simulink model "JointSpaceControl_BestInertia"  (R2013a)
settings: Solver=ode3  StartTime=0.0  StopTime=sim_end  FixedStep=0.004  MaxStep=0.008  RelTol=1e-3
PreLoadFcn:
  | Initialization
InitFcn:
  | Initialization
values from neighbouring files (symbols this model uses):
  a_max = [27 27 27 27 27 27]    [Initialization.m]
  dq_0 = qd_actual.signals.values(1,:)    [Initialization.m]
  K_0 = [K0_11, zeros(3,3); zeros(3,3),omega_P_small^2*eye(3,3)]    [Initialization.m]    (also in Plot_PD_Estimation.m)
  K_1 = [K1_11, zeros(3,3); zeros(3,3),2*omega_D_small*eye(3,3)]    [Initialization.m]    (also in Plot_PD_Estimation.m)
  q_0 = q_actual.signals.values(1,:)    [Initialization.m]
  q_max = 2*pi*ones(1,6)    [Initialization.m]
  q_min = -2*pi*ones(1,6)    [Initialization.m]
  torque_max = [150 150 150 28 28 28]    [Initialization.m]
  v_max = 3.4*ones(1,6)    [Initialization.m]
libraries: dsparch4 x30, simulink x2
(part 3 of 3)

== matlab function JointSpaceControl_BestInertia/Forward & Velocity Kinematics Joint -> Tool Geometric Jacobian/J_a ==
  data: J_a output; q input; theta input; phi input; psi input
function J_a     = Analytical_Jacobian(q, theta, phi, psi)
% ANALYTICAL JACOBIAN - Jacobian from Base to Tool.
%  Calculates the analytical Jacobian, based on the Euler angle transform
%  representation.

theta_1 = q(1);
theta_2 = q(2);
theta_3 = q(3);
theta_4 = q(4);
theta_5 = q(5);
theta_6 = q(6);

J = [(109*cos(theta_1))/1000 + (41*cos(theta_1)*cos(theta_5))/500 + ...
        (17*cos(theta_2)*sin(theta_1))/40 - ...
        (93*cos(theta_4)*(cos(theta_2)*sin(theta_1)*sin(theta_3) + ...
        cos(theta_3)*sin(theta_1)*sin(theta_2)))/1000 + ...
        (93*sin(theta_4)*(sin(theta_1)*sin(theta_2)*sin(theta_3) - ...
        cos(theta_2)*cos(theta_3)*sin(theta_1)))/1000 - ...
        (41*sin(theta_5)*(cos(theta_4)*(sin(theta_1)*sin(theta_2)*sin(theta_3) - ...
        cos(theta_2)*cos(theta_3)*sin(theta_1)) + ...
        sin(theta_4)*(cos(theta_2)*sin(theta_1)*sin(theta_3) + ...
        cos(theta_3)*sin(theta_1)*sin(theta_2))))/500 - ...
        (39243*sin(theta_1)*sin(theta_2)*sin(theta_3))/100000 + ...
        (39243*cos(theta_2)*cos(theta_3)*sin(theta_1))/100000, ...
        ...
        (17*cos(theta_1)*sin(theta_2))/40 - ...
        (93*cos(theta_4)*(cos(theta_1)*sin(theta_2)*sin(theta_3) - ...
        cos(theta_1)*cos(theta_2)*cos(theta_3)))/1000 - ...
        (93*sin(theta_4)*(cos(theta_1)*cos(theta_2)*sin(theta_3) + ...
        cos(theta_1)*cos(theta_3)*sin(theta_2)))/1000 + ...
        (41*sin(theta_5)*(cos(theta_4)*(cos(theta_1)*cos(theta_2)*sin(theta_3) + ...
        cos(theta_1)*cos(theta_3)*sin(theta_2)) - ...
        sin(theta_4)*(cos(theta_1)*sin(theta_2)*sin(theta_3) - ...
        cos(theta_1)*cos(theta_2)*cos(theta_3))))/500 + ...
        (39243*cos(theta_1)*cos(theta_2)*sin(theta_3))/100000 + ...
        (39243*cos(theta_1)*cos(theta_3)*sin(theta_2))/100000, ...
        ...
        (41*sin(theta_5)*(cos(theta_4)*(cos(theta_1)*cos(theta_2)*sin(theta_3) + ...
        cos(theta_1)*cos(theta_3)*sin(theta_2)) - ...
        sin(theta_4)*(cos(theta_1)*sin(theta_2)*sin(theta_3) - ...
        cos(theta_1)*cos(theta_2)*cos(theta_3))))/500 - ...
        (93*sin(theta_4)*(cos(theta_1)*cos(theta_2)*sin(theta_3) + ...
        cos(theta_1)*cos(theta_3)*sin(theta_2)))/1000 - ...
        (93*cos(theta_4)*(cos(theta_1)*sin(theta_2)*sin(theta_3) - ...
        cos(theta_1)*cos(theta_2)*cos(theta_3)))/1000 + ...
        (39243*cos(theta_1)*cos(theta_2)*sin(theta_3))/100000 + ...
        (39243*cos(theta_1)*cos(theta_3)*sin(theta_2))/100000, ...
        ...
        (41*sin(theta_5)*(cos(theta_4)*(cos(theta_1)*cos(theta_2)*sin(theta_3) + ...
        cos(theta_1)*cos(theta_3)*sin(theta_2)) - ...
        sin(theta_4)*(cos(theta_1)*sin(theta_2)*sin(theta_3) - ...
        cos(theta_1)*cos(theta_2)*cos(theta_3))))/500 - ...
        (93*sin(theta_4)*(cos(theta_1)*cos(theta_2)*sin(theta_3) + ...
        cos(theta_1)*cos(theta_3)*sin(theta_2)))/1000 - ...
        (93*cos(theta_4)*(cos(theta_1)*sin(theta_2)*sin(theta_3) - ...
        cos(theta_1)*cos(theta_2)*cos(theta_3)))/1000, ...
        ...
        (41*cos(theta_5)*(cos(theta_4)*(cos(theta_1)*sin(theta_2)*sin(theta_3) - ...
        cos(theta_1)*cos(theta_2)*cos(theta_3)) + ...
        sin(theta_4)*(cos(theta_1)*cos(theta_2)*sin(theta_3) + ...
        cos(theta_1)*cos(theta_3)*sin(theta_2))))/500 - ...
        (41*sin(theta_1)*sin(theta_5))/500,... 
        ...
        0; ...
   (109*sin(theta_1))/1000 - (17*cos(theta_1)*cos(theta_2))/40 + ...
        (41*cos(theta_5)*sin(theta_1))/500 + ...
        (93*cos(theta_4)*(cos(theta_1)*cos(theta_2)*sin(theta_3) + ...
        cos(theta_1)*cos(theta_3)*sin(theta_2)))/1000 - ...
        (93*sin(theta_4)*(cos(theta_1)*sin(theta_2)*sin(theta_3) - ... 
        cos(theta_1)*cos(theta_2)*cos(theta_3)))/1000 + ...
        (41*sin(theta_5)*(cos(theta_4)*(cos(theta_1)*sin(theta_2)*sin(theta_3) - ...
        cos(theta_1)*cos(theta_2)*cos(theta_3)) + ...
        sin(theta_4)*(cos(theta_1)*cos(theta_2)*sin(theta_3) + ...
        cos(theta_1)*cos(theta_3)*sin(theta_2))))/500 + ...
        (39243*cos(theta_1)*sin(theta_2)*sin(theta_3))/100000 - ...
        (39243*cos(theta_1)*cos(theta_2)*cos(theta_3))/100000, ...
        ...
        (17*sin(theta_1)*sin(theta_2))/40 - ...
        (93*cos(theta_4)*(sin(theta_1)*sin(theta_2)*sin(theta_3) - ...
        cos(theta_2)*cos(theta_3)*sin(theta_1)))/1000 - ...
        (93*sin(theta_4)*(cos(theta_2)*sin(theta_1)*sin(theta_3) + ...
        cos(theta_3)*sin(theta_1)*sin(theta_2)))/1000 + ...
        (41*sin(theta_5)*(cos(theta_4)*(cos(theta_2)*sin(theta_1)*sin(theta_3) + ...
        cos(theta_3)*sin(theta_1)*sin(theta_2)) - ...
        sin(theta_4)*(sin(theta_1)*sin(theta_2)*sin(theta_3) - ...
        cos(theta_2)*cos(theta_3)*sin(theta_1))))/500 + ...
        (39243*cos(theta_2)*sin(theta_1)*sin(theta_3))/100000 + ...
        (39243*cos(theta_3)*sin(theta_1)*sin(theta_2))/100000, ...
        ...
        (41*sin(theta_5)*(cos(theta_4)*(cos(theta_2)*sin(theta_1)*sin(theta_3) + ...
        cos(theta_3)*sin(theta_1)*sin(theta_2)) - ...
        sin(theta_4)*(sin(theta_1)*sin(theta_2)*sin(theta_3) - ...
        cos(theta_2)*cos(theta_3)*sin(theta_1))))/500 - ...
        (93*sin(theta_4)*(cos(theta_2)*sin(theta_1)*sin(theta_3) + ...
        cos(theta_3)*sin(theta_1)*sin(theta_2)))/1000 - ...
        (93*cos(theta_4)*(sin(theta_1)*sin(theta_2)*sin(theta_3) - ...
        cos(theta_2)*cos(theta_3)*sin(theta_1)))/1000 + ...
        (39243*cos(theta_2)*sin(theta_1)*sin(theta_3))/100000 + ...
        (39243*cos(theta_3)*sin(theta_1)*sin(theta_2))/100000, ...
        ...
        (41*sin(theta_5)*(cos(theta_4)*(cos(theta_2)*sin(theta_1)*sin(theta_3) + ...
        cos(theta_3)*sin(theta_1)*sin(theta_2)) - ...
        sin(theta_4)*(sin(theta_1)*sin(theta_2)*sin(theta_3) - ...
        cos(theta_2)*cos(theta_3)*sin(theta_1))))/500 - ...
        (93*sin(theta_4)*(cos(theta_2)*sin(theta_1)*sin(theta_3) + ...
        cos(theta_3)*sin(theta_1)*sin(theta_2)))/1000 - ...
        (93*cos(theta_4)*(sin(theta_1)*sin(theta_2)*sin(theta_3) - ...
        cos(theta_2)*cos(theta_3)*sin(theta_1)))/1000, ...
        ...
        (41*cos(theta_1)*sin(theta_5))/500 + ...
        (41*cos(theta_5)*(cos(theta_4)*(sin(theta_1)*sin(theta_2)*sin(theta_3) - ...
        cos(theta_2)*cos(theta_3)*sin(theta_1)) + ...
        sin(theta_4)*(cos(theta_2)*sin(theta_1)*sin(theta_3) + ...
        cos(theta_3)*sin(theta_1)*sin(theta_2))))/500, ...
        ...
        0; ...
    0, ...
        ...
        (39243*sin(theta_2)*sin(theta_3))/100000 - ...
        (39243*cos(theta_2)*cos(theta_3))/100000 - ...
        (17*cos(theta_2))/40 - ...
        (41*sin(theta_5)*(cos(theta_4)*(cos(theta_2)*cos(theta_3) - ...
        sin(theta_2)*sin(theta_3)) - sin(theta_4)*(cos(theta_2)*sin(theta_3) + ...
        cos(theta_3)*sin(theta_2))))/500 + ...
        (93*cos(theta_4)*(cos(theta_2)*sin(theta_3) + ...
        cos(theta_3)*sin(theta_2)))/1000 + ...
        (93*sin(theta_4)*(cos(theta_2)*cos(theta_3) - sin(theta_2)*sin(theta_3)))/1000,...
        ...
        (39243*sin(theta_2)*sin(theta_3))/100000 - ...
        (39243*cos(theta_2)*cos(theta_3))/100000 - ...
        (41*sin(theta_5)*(cos(theta_4)*(cos(theta_2)*cos(theta_3) - ...
        sin(theta_2)*sin(theta_3)) - sin(theta_4)*(cos(theta_2)*sin(theta_3) + ...
        cos(theta_3)*sin(theta_2))))/500 + (93*cos(theta_4)*(cos(theta_2)*sin(theta_3) + ...
        cos(theta_3)*sin(theta_2)))/1000 + (93*sin(theta_4)*(cos(theta_2)*cos(theta_3) - ...
        sin(theta_2)*sin(theta_3)))/1000, ...
        ...
        (93*cos(theta_4)*(cos(theta_2)*sin(theta_3) + cos(theta_3)*sin(theta_2)))/1000 - ...
        (41*sin(theta_5)*(cos(theta_4)*(cos(theta_2)*cos(theta_3) - ...
        sin(theta_2)*sin(theta_3)) - sin(theta_4)*(cos(theta_2)*sin(theta_3) + ...
        cos(theta_3)*sin(theta_2))))/500 + (93*sin(theta_4)*(cos(theta_2)*cos(theta_3) - ...
        sin(theta_2)*sin(theta_3)))/1000,  ...
        ...
        -(41*cos(theta_5)*(cos(theta_4)*(cos(theta_2)*sin(theta_3) + ...
        cos(theta_3)*sin(theta_2)) + sin(theta_4)*(cos(theta_2)*cos(theta_3) - ...
        sin(theta_2)*sin(theta_3))))/500,  ...
        ...
        0; ...
    0, ...
        ...
        sin(theta_1), ...
        ...
        sin(theta_1), ...
        ...
        sin(theta_1), ...
        ...
        cos(theta_4)*(cos(theta_1)*cos(theta_2)*sin(theta_3) + ...
        cos(theta_1)*cos(theta_3)*sin(theta_2)) - ...
        sin(theta_4)*(cos(theta_1)*sin(theta_2)*sin(theta_3) - ...
        cos(theta_1)*cos(theta_2)*cos(theta_3)), ...
        ...
        cos(theta_5)*sin(theta_1) + ...
        sin(theta_5)*(cos(theta_4)*(cos(theta_1)*sin(theta_2)*sin(theta_3) - ...
        cos(theta_1)*cos(theta_2)*cos(theta_3)) + ...
        sin(theta_4)*(cos(theta_1)*cos(theta_2)*sin(theta_3) + ...
        cos(theta_1)*cos(theta_3)*sin(theta_2)));...
    0, ...
        ...
        -cos(theta_1), ...
        ...
        -cos(theta_1), ...
        ...
        -cos(theta_1), ...
        ...
        cos(theta_4)*(cos(theta_2)*sin(theta_1)*sin(theta_3) + ...
        cos(theta_3)*sin(theta_1)*sin(theta_2)) - ...
        sin(theta_4)*(sin(theta_1)*sin(theta_2)*sin(theta_3) - ...
        cos(theta_2)*cos(theta_3)*sin(theta_1)), ...
        ...
        sin(theta_5)*(cos(theta_4)*(sin(theta_1)*sin(theta_2)*sin(theta_3) - ...
        cos(theta_2)*cos(theta_3)*sin(theta_1)) + ...
        sin(theta_4)*(cos(theta_2)*sin(theta_1)*sin(theta_3) + ...
        cos(theta_3)*sin(theta_1)*sin(theta_2))) - cos(theta_1)*cos(theta_5);
    1, ...
        ...
        0, ...
        ...
        0, ...
        ...
        0, ...
        ...
        sin(theta_4)*(cos(theta_2)*sin(theta_3) + cos(theta_3)*sin(theta_2)) - ...
        cos(theta_4)*(cos(theta_2)*cos(theta_3) - sin(theta_2)*sin(theta_3)),...
        ...
        -sin(theta_5)*(cos(theta_4)*(cos(theta_2)*sin(theta_3) + ...
        cos(theta_3)*sin(theta_2)) + sin(theta_4)*(cos(theta_2)*cos(theta_3) - ...
        sin(theta_2)*sin(theta_3)));];

    B_alpha = [cos(psi)*sin(theta), -sin(psi), 0; ...
               sin(psi)*sin(theta), cos(psi), 0; ...
               cos(theta), 0, 1];
    Transf = [eye(3,3), zeros(3,3); zeros(3,3), inv(B_alpha)];
    J_a = Transf*J;

end

== matlab function JointSpaceControl_BestInertia/Forward & Velocity Kinematics Joint -> Tool Geometric Jacobian/End-Effector -> Joints/base_tool_transformation_matrix2 ==
  data: d output; q input; R output
function [d, R]   = base_tool_transformation(q)
% BASE_TOOL_TRANSFORMATION - Transformationmatrix from Base to Tool.
%  Calculates the Base-Tool Transformation matrix based on the current
%  joint positions and returns the rotation matrix and the displacement
%  vector.

theta1 = q(1);
theta2 = q(2);
theta3 = q(3);
theta4 = q(4);
theta5 = q(5);
theta6 = q(6);

theta_1 = theta1;
theta_2 = theta2;
theta_3 = theta3;
theta_4 = theta4;
theta_5 = theta5;
theta_6 = theta6;

% With transformation to accelerometer
T = [[   cos(theta_6)*(sin(theta_1)*sin(theta_5) - cos(theta_5)*(cos(theta_4)*(cos(theta_1)*sin(theta_2)*sin(theta_3) - cos(theta_1)*cos(theta_2)*cos(theta_3)) + sin(theta_4)*(cos(theta_1)*cos(theta_2)*sin(theta_3) + cos(theta_1)*cos(theta_3)*sin(theta_2)))) - sin(theta_6)*(cos(theta_4)*(cos(theta_1)*cos(theta_2)*sin(theta_3) + cos(theta_1)*cos(theta_3)*sin(theta_2)) - sin(theta_4)*(cos(theta_1)*sin(theta_2)*sin(theta_3) - cos(theta_1)*cos(theta_2)*cos(theta_3))), - sin(theta_6)*(sin(theta_1)*sin(theta_5) - cos(theta_5)*(cos(theta_4)*(cos(theta_1)*sin(theta_2)*sin(theta_3) - cos(theta_1)*cos(theta_2)*cos(theta_3)) + sin(theta_4)*(cos(theta_1)*cos(theta_2)*sin(theta_3) + cos(theta_1)*cos(theta_3)*sin(theta_2)))) - cos(theta_6)*(cos(theta_4)*(cos(theta_1)*cos(theta_2)*sin(theta_3) + cos(theta_1)*cos(theta_3)*sin(theta_2)) - sin(theta_4)*(cos(theta_1)*sin(theta_2)*sin(theta_3) - cos(theta_1)*cos(theta_2)*cos(theta_3))), cos(theta_5)*sin(theta_1) + sin(theta_5)*(cos(theta_4)*(cos(theta_1)*sin(theta_2)*sin(theta_3) - cos(theta_1)*cos(theta_2)*cos(theta_3)) + sin(theta_4)*(cos(theta_1)*cos(theta_2)*sin(theta_3) + cos(theta_1)*cos(theta_3)*sin(theta_2))), (109*sin(theta_1))/1000 - (17*cos(theta_1)*cos(theta_2))/40 + (183*cos(theta_5)*sin(theta_1))/2000 + (347*cos(theta_6)*(sin(theta_1)*sin(theta_5) - cos(theta_5)*(cos(theta_4)*(cos(theta_1)*sin(theta_2)*sin(theta_3) - cos(theta_1)*cos(theta_2)*cos(theta_3)) + sin(theta_4)*(cos(theta_1)*cos(theta_2)*sin(theta_3) + cos(theta_1)*cos(theta_3)*sin(theta_2)))))/20000 + (93*cos(theta_4)*(cos(theta_1)*cos(theta_2)*sin(theta_3) + cos(theta_1)*cos(theta_3)*sin(theta_2)))/1000 - (121*sin(theta_6)*(sin(theta_1)*sin(theta_5) - cos(theta_5)*(cos(theta_4)*(cos(theta_1)*sin(theta_2)*sin(theta_3) - cos(theta_1)*cos(theta_2)*cos(theta_3)) + sin(theta_4)*(cos(theta_1)*cos(theta_2)*sin(theta_3) + cos(theta_1)*cos(theta_3)*sin(theta_2)))))/20000 - (93*sin(theta_4)*(cos(theta_1)*sin(theta_2)*sin(theta_3) - cos(theta_1)*cos(theta_2)*cos(theta_3)))/1000 - (121*cos(theta_6)*(cos(theta_4)*(cos(theta_1)*cos(theta_2)*sin(theta_3) + cos(theta_1)*cos(theta_3)*sin(theta_2)) - sin(theta_4)*(cos(theta_1)*sin(theta_2)*sin(theta_3) - cos(theta_1)*cos(theta_2)*cos(theta_3))))/20000 + (183*sin(theta_5)*(cos(theta_4)*(cos(theta_1)*sin(theta_2)*sin(theta_3) - cos(theta_1)*cos(theta_2)*cos(theta_3)) + sin(theta_4)*(cos(theta_1)*cos(theta_2)*sin(theta_3) + cos(theta_1)*cos(theta_3)*sin(theta_2))))/2000 - (347*sin(theta_6)*(cos(theta_4)*(cos(theta_1)*cos(theta_2)*sin(theta_3) + cos(theta_1)*cos(theta_3)*sin(theta_2)) - sin(theta_4)*(cos(theta_1)*sin(theta_2)*sin(theta_3) - cos(theta_1)*cos(theta_2)*cos(theta_3))))/20000 + (39243*cos(theta_1)*sin(theta_2)*sin(theta_3))/100000 - (39243*cos(theta_1)*cos(theta_2)*cos(theta_3))/100000]; 
    [ - cos(theta_6)*(cos(theta_1)*sin(theta_5) + cos(theta_5)*(cos(theta_4)*(sin(theta_1)*sin(theta_2)*sin(theta_3) - cos(theta_2)*cos(theta_3)*sin(theta_1)) + sin(theta_4)*(cos(theta_2)*sin(theta_1)*sin(theta_3) + cos(theta_3)*sin(theta_1)*sin(theta_2)))) - sin(theta_6)*(cos(theta_4)*(cos(theta_2)*sin(theta_1)*sin(theta_3) + cos(theta_3)*sin(theta_1)*sin(theta_2)) - sin(theta_4)*(sin(theta_1)*sin(theta_2)*sin(theta_3) - cos(theta_2)*cos(theta_3)*sin(theta_1))),   sin(theta_6)*(cos(theta_1)*sin(theta_5) + cos(theta_5)*(cos(theta_4)*(sin(theta_1)*sin(theta_2)*sin(theta_3) - cos(theta_2)*cos(theta_3)*sin(theta_1)) + sin(theta_4)*(cos(theta_2)*sin(theta_1)*sin(theta_3) + cos(theta_3)*sin(theta_1)*sin(theta_2)))) - cos(theta_6)*(cos(theta_4)*(cos(theta_2)*sin(theta_1)*sin(theta_3) + cos(theta_3)*sin(theta_1)*sin(theta_2)) - sin(theta_4)*(sin(theta_1)*sin(theta_2)*sin(theta_3) - cos(theta_2)*cos(theta_3)*sin(theta_1))), sin(theta_5)*(cos(theta_4)*(sin(theta_1)*sin(theta_2)*sin(theta_3) - cos(theta_2)*cos(theta_3)*sin(theta_1)) + sin(theta_4)*(cos(theta_2)*sin(theta_1)*sin(theta_3) + cos(theta_3)*sin(theta_1)*sin(theta_2))) - cos(theta_1)*cos(theta_5), (93*cos(theta_4)*(cos(theta_2)*sin(theta_1)*sin(theta_3) + cos(theta_3)*sin(theta_1)*sin(theta_2)))/1000 - (183*cos(theta_1)*cos(theta_5))/2000 - (17*cos(theta_2)*sin(theta_1))/40 - (109*cos(theta_1))/1000 - (347*cos(theta_6)*(cos(theta_1)*sin(theta_5) + cos(theta_5)*(cos(theta_4)*(sin(theta_1)*sin(theta_2)*sin(theta_3) - cos(theta_2)*cos(theta_3)*sin(theta_1)) + sin(theta_4)*(cos(theta_2)*sin(theta_1)*sin(theta_3) + cos(theta_3)*sin(theta_1)*sin(theta_2)))))/20000 - (93*sin(theta_4)*(sin(theta_1)*sin(theta_2)*sin(theta_3) - cos(theta_2)*cos(theta_3)*sin(theta_1)))/1000 + (121*sin(theta_6)*(cos(theta_1)*sin(theta_5) + cos(theta_5)*(cos(theta_4)*(sin(theta_1)*sin(theta_2)*sin(theta_3) - cos(theta_2)*cos(theta_3)*sin(theta_1)) + sin(theta_4)*(cos(theta_2)*sin(theta_1)*sin(theta_3) + cos(theta_3)*sin(theta_1)*sin(theta_2)))))/20000 - (121*cos(theta_6)*(cos(theta_4)*(cos(theta_2)*sin(theta_1)*sin(theta_3) + cos(theta_3)*sin(theta_1)*sin(theta_2)) - sin(theta_4)*(sin(theta_1)*sin(theta_2)*sin(theta_3) - cos(theta_2)*cos(theta_3)*sin(theta_1))))/20000 + (183*sin(theta_5)*(cos(theta_4)*(sin(theta_1)*sin(theta_2)*sin(theta_3) - cos(theta_2)*cos(theta_3)*sin(theta_1)) + sin(theta_4)*(cos(theta_2)*sin(theta_1)*sin(theta_3) + cos(theta_3)*sin(theta_1)*sin(theta_2))))/2000 - (347*sin(theta_6)*(cos(theta_4)*(cos(theta_2)*sin(theta_1)*sin(theta_3) + cos(theta_3)*sin(theta_1)*sin(theta_2)) - sin(theta_4)*(sin(theta_1)*sin(theta_2)*sin(theta_3) - cos(theta_2)*cos(theta_3)*sin(theta_1))))/20000 + (39243*sin(theta_1)*sin(theta_2)*sin(theta_3))/100000 - (39243*cos(theta_2)*cos(theta_3)*sin(theta_1))/100000]; 
    [                                                                                                                                         sin(theta_6)*(cos(theta_4)*(cos(theta_2)*cos(theta_3) - sin(theta_2)*sin(theta_3)) - sin(theta_4)*(cos(theta_2)*sin(theta_3) + cos(theta_3)*sin(theta_2))) + cos(theta_5)*cos(theta_6)*(cos(theta_4)*(cos(theta_2)*sin(theta_3) + cos(theta_3)*sin(theta_2)) + sin(theta_4)*(cos(theta_2)*cos(theta_3) - sin(theta_2)*sin(theta_3))),                                                                                                                                         cos(theta_6)*(cos(theta_4)*(cos(theta_2)*cos(theta_3) - sin(theta_2)*sin(theta_3)) - sin(theta_4)*(cos(theta_2)*sin(theta_3) + cos(theta_3)*sin(theta_2))) - cos(theta_5)*sin(theta_6)*(cos(theta_4)*(cos(theta_2)*sin(theta_3) + cos(theta_3)*sin(theta_2)) + sin(theta_4)*(cos(theta_2)*cos(theta_3) - sin(theta_2)*sin(theta_3))),                                                                                -sin(theta_5)*(cos(theta_4)*(cos(theta_2)*sin(theta_3) + cos(theta_3)*sin(theta_2)) + sin(theta_4)*(cos(theta_2)*cos(theta_3) - sin(theta_2)*sin(theta_3))),                                                                                                                                                                                                                                                                                                                                                                                                                                                                                  (121*cos(theta_6)*(cos(theta_4)*(cos(theta_2)*cos(theta_3) - sin(theta_2)*sin(theta_3)) - sin(theta_4)*(cos(theta_2)*sin(theta_3) + cos(theta_3)*sin(theta_2))))/20000 - (39243*cos(theta_2)*sin(theta_3))/100000 - (39243*cos(theta_3)*sin(theta_2))/100000 - (17*sin(theta_2))/40 - (183*sin(theta_5)*(cos(theta_4)*(cos(theta_2)*sin(theta_3) + cos(theta_3)*sin(theta_2)) + sin(theta_4)*(cos(theta_2)*cos(theta_3) - sin(theta_2)*sin(theta_3))))/2000 + (347*sin(theta_6)*(cos(theta_4)*(cos(theta_2)*cos(theta_3) - sin(theta_2)*sin(theta_3)) - sin(theta_4)*(cos(theta_2)*sin(theta_3) + cos(theta_3)*sin(theta_2))))/20000 - (93*cos(theta_4)*(cos(theta_2)*cos(theta_3) - sin(theta_2)*sin(theta_3)))/1000 + (93*sin(theta_4)*(cos(theta_2)*sin(theta_3) + cos(theta_3)*sin(theta_2)))/1000 + (347*cos(theta_5)*cos(theta_6)*(cos(theta_4)*(cos(theta_2)*sin(theta_3) + cos(theta_3)*sin(theta_2)) + sin(theta_4)*(cos(theta_2)*cos(theta_3) - sin(theta_2)*sin(theta_3))))/20000 - (121*cos(theta_5)*sin(theta_6)*(cos(theta_4)*(cos(theta_2)*sin(theta_3) + cos(theta_3)*sin(theta_2)) + sin(theta_4)*(cos(theta_2)*cos(theta_3) - sin(theta_2)*sin(theta_3))))/20000 + 223/2500]; 
    [                                                                                                                                                                                                                                                                                                                                                                                                                                                                            0,                                                                                                                                                                                                                                                                                                                                                                                                                                                                            0,                                                                                                                                                                                                                                          0,                                                                                                                                                                                                                                                                                                                                                                                                                                                                                                                                                                                                                                                                                                                                                                                                                                                                                                                                                                                                                                                                                                                                                                                                                                                                                                                                                                                                                                                                                                                                                                                                                                                                              1]];


% T =  [[cos(theta_6)*(sin(theta_1)*sin(theta_5) - cos(theta_5)*(cos(theta_4)*(cos(theta_1)*sin(theta_2)*sin(theta_3) - cos(theta_1)*cos(theta_2)*cos(theta_3)) + sin(theta_4)*(cos(theta_1)*cos(theta_2)*sin(theta_3) + cos(theta_1)*cos(theta_3)*sin(theta_2)))) - sin(theta_6)*(cos(theta_4)*(cos(theta_1)*cos(theta_2)*sin(theta_3) + cos(theta_1)*cos(theta_3)*sin(theta_2)) - sin(theta_4)*(cos(theta_1)*sin(theta_2)*sin(theta_3) - cos(theta_1)*cos(theta_2)*cos(theta_3))), - sin(theta_6)*(sin(theta_1)*sin(theta_5) - cos(theta_5)*(cos(theta_4)*(cos(theta_1)*sin(theta_2)*sin(theta_3) - cos(theta_1)*cos(theta_2)*cos(theta_3)) + sin(theta_4)*(cos(theta_1)*cos(theta_2)*sin(theta_3) + cos(theta_1)*cos(theta_3)*sin(theta_2)))) - cos(theta_6)*(cos(theta_4)*(cos(theta_1)*cos(theta_2)*sin(theta_3) + cos(theta_1)*cos(theta_3)*sin(theta_2)) - sin(theta_4)*(cos(theta_1)*sin(theta_2)*sin(theta_3) - cos(theta_1)*cos(theta_2)*cos(theta_3))), cos(theta_5)*sin(theta_1) + sin(theta_5)*(cos(theta_4)*(cos(theta_1)*sin(theta_2)*sin(theta_3) - cos(theta_1)*cos(theta_2)*cos(theta_3)) + sin(theta_4)*(cos(theta_1)*cos(theta_2)*sin(theta_3) + cos(theta_1)*cos(theta_3)*sin(theta_2))), (109*sin(theta_1))/1000 - (17*cos(theta_1)*cos(theta_2))/40 + (41*cos(theta_5)*sin(theta_1))/500 + (93*cos(theta_4)*(cos(theta_1)*cos(theta_2)*sin(theta_3) + cos(theta_1)*cos(theta_3)*sin(theta_2)))/1000 - (93*sin(theta_4)*(cos(theta_1)*sin(theta_2)*sin(theta_3) - cos(theta_1)*cos(theta_2)*cos(theta_3)))/1000 + (41*sin(theta_5)*(cos(theta_4)*(cos(theta_1)*sin(theta_2)*sin(theta_3) - cos(theta_1)*cos(theta_2)*cos(theta_3)) + sin(theta_4)*(cos(theta_1)*cos(theta_2)*sin(theta_3) + cos(theta_1)*cos(theta_3)*sin(theta_2))))/500 + (39243*cos(theta_1)*sin(theta_2)*sin(theta_3))/100000 - (39243*cos(theta_1)*cos(theta_2)*cos(theta_3))/100000];
%      [ - cos(theta_6)*(cos(theta_1)*sin(theta_5) + cos(theta_5)*(cos(theta_4)*(sin(theta_1)*sin(theta_2)*sin(theta_3) - cos(theta_2)*cos(theta_3)*sin(theta_1)) + sin(theta_4)*(cos(theta_2)*sin(theta_1)*sin(theta_3) + cos(theta_3)*sin(theta_1)*sin(theta_2)))) - sin(theta_6)*(cos(theta_4)*(cos(theta_2)*sin(theta_1)*sin(theta_3) + cos(theta_3)*sin(theta_1)*sin(theta_2)) - sin(theta_4)*(sin(theta_1)*sin(theta_2)*sin(theta_3) - cos(theta_2)*cos(theta_3)*sin(theta_1))),   sin(theta_6)*(cos(theta_1)*sin(theta_5) + cos(theta_5)*(cos(theta_4)*(sin(theta_1)*sin(theta_2)*sin(theta_3) - cos(theta_2)*cos(theta_3)*sin(theta_1)) + sin(theta_4)*(cos(theta_2)*sin(theta_1)*sin(theta_3) + cos(theta_3)*sin(theta_1)*sin(theta_2)))) - cos(theta_6)*(cos(theta_4)*(cos(theta_2)*sin(theta_1)*sin(theta_3) + cos(theta_3)*sin(theta_1)*sin(theta_2)) - sin(theta_4)*(sin(theta_1)*sin(theta_2)*sin(theta_3) - cos(theta_2)*cos(theta_3)*sin(theta_1))), sin(theta_5)*(cos(theta_4)*(sin(theta_1)*sin(theta_2)*sin(theta_3) - cos(theta_2)*cos(theta_3)*sin(theta_1)) + sin(theta_4)*(cos(theta_2)*sin(theta_1)*sin(theta_3) + cos(theta_3)*sin(theta_1)*sin(theta_2))) - cos(theta_1)*cos(theta_5), (93*cos(theta_4)*(cos(theta_2)*sin(theta_1)*sin(theta_3) + cos(theta_3)*sin(theta_1)*sin(theta_2)))/1000 - (41*cos(theta_1)*cos(theta_5))/500 - (17*cos(theta_2)*sin(theta_1))/40 - (109*cos(theta_1))/1000 - (93*sin(theta_4)*(sin(theta_1)*sin(theta_2)*sin(theta_3) - cos(theta_2)*cos(theta_3)*sin(theta_1)))/1000 + (41*sin(theta_5)*(cos(theta_4)*(sin(theta_1)*sin(theta_2)*sin(theta_3) - cos(theta_2)*cos(theta_3)*sin(theta_1)) + sin(theta_4)*(cos(theta_2)*sin(theta_1)*sin(theta_3) + cos(theta_3)*sin(theta_1)*sin(theta_2))))/500 + (39243*sin(theta_1)*sin(theta_2)*sin(theta_3))/100000 - (39243*cos(theta_2)*cos(theta_3)*sin(theta_1))/100000];
%      [                                                                                                                                         sin(theta_6)*(cos(theta_4)*(cos(theta_2)*cos(theta_3) - sin(theta_2)*sin(theta_3)) - sin(theta_4)*(cos(theta_2)*sin(theta_3) + cos(theta_3)*sin(theta_2))) + cos(theta_5)*cos(theta_6)*(cos(theta_4)*(cos(theta_2)*sin(theta_3) + cos(theta_3)*sin(theta_2)) + sin(theta_4)*(cos(theta_2)*cos(theta_3) - sin(theta_2)*sin(theta_3))),                                                                                                                                         cos(theta_6)*(cos(theta_4)*(cos(theta_2)*cos(theta_3) - sin(theta_2)*sin(theta_3)) - sin(theta_4)*(cos(theta_2)*sin(theta_3) + cos(theta_3)*sin(theta_2))) - cos(theta_5)*sin(theta_6)*(cos(theta_4)*(cos(theta_2)*sin(theta_3) + cos(theta_3)*sin(theta_2)) + sin(theta_4)*(cos(theta_2)*cos(theta_3) - sin(theta_2)*sin(theta_3))),                                                                                -sin(theta_5)*(cos(theta_4)*(cos(theta_2)*sin(theta_3) + cos(theta_3)*sin(theta_2)) + sin(theta_4)*(cos(theta_2)*cos(theta_3) - sin(theta_2)*sin(theta_3))),                                                                                                                                                                                                    (93*sin(theta_4)*(cos(theta_2)*sin(theta_3) + cos(theta_3)*sin(theta_2)))/1000 - (39243*cos(theta_2)*sin(theta_3))/100000 - (39243*cos(theta_3)*sin(theta_2))/100000 - (41*sin(theta_5)*(cos(theta_4)*(cos(theta_2)*sin(theta_3) + cos(theta_3)*sin(theta_2)) + sin(theta_4)*(cos(theta_2)*cos(theta_3) - sin(theta_2)*sin(theta_3))))/500 - (93*cos(theta_4)*(cos(theta_2)*cos(theta_3) - sin(theta_2)*sin(theta_3)))/1000 - (17*sin(theta_2))/40 + 223/2500];
%      [                                                                                                                                                                                                                                                                                                                                                                                                                                                                            0,                                                                                                                                                                                                                                                                                                                                                                                                                                                                            0,                                                                                                                                                                                                                                          0,                                                                                                                                                                                                                                                                                                                                                                                                                                                                                                                                                                                                                                                                1]];


% 
% T = [(((cos(theta1) * cos(theta2) * cos(theta3) - cos(theta1) * sin(theta2) ...
%     * sin(theta3)) * cos(theta4) + (-cos(theta1) * cos(theta2) * sin(theta3) ...
%     - cos(theta1) * sin(theta2) * cos(theta3)) * sin(theta4)) * cos(theta5) ...
%     + sin(theta1) * sin(theta5)) * cos(theta6) + (-(cos(theta1) * cos(theta2) ...
%     * cos(theta3) - cos(theta1) * sin(theta2) * sin(theta3)) * sin(theta4) + ...
%     (-cos(theta1) * cos(theta2) * sin(theta3) - cos(theta1) * sin(theta2) * ...
%     cos(theta3)) * cos(theta4)) * sin(theta6) -(((cos(theta1) * cos(theta2) * ...
%     cos(theta3) - cos(theta1) * sin(theta2) * sin(theta3)) * cos(theta4) + ...
%     (-cos(theta1) * cos(theta2) * sin(theta3) - cos(theta1) * sin(theta2) * ...
%     cos(theta3)) * sin(theta4)) * cos(theta5) + sin(theta1) * sin(theta5)) * ...
%     sin(theta6) + (-(cos(theta1) * cos(theta2) * cos(theta3) - cos(theta1) * ...
%     sin(theta2) * sin(theta3)) * sin(theta4) + (-cos(theta1) * cos(theta2) * ...
%     sin(theta3) - cos(theta1) * sin(theta2) * cos(theta3)) * cos(theta4)) * ...
%     cos(theta6) -((cos(theta1) * cos(theta2) * cos(theta3) - cos(theta1) * ...
%     sin(theta2) * sin(theta3)) * cos(theta4) + (-cos(theta1) * cos(theta2) * ...
%     sin(theta3) - cos(theta1) * sin(theta2) * cos(theta3)) * sin(theta4)) * ...
%     sin(theta5) + sin(theta1) * cos(theta5) -0.082 * ((cos(theta1) * ...
%     cos(theta2) * cos(theta3) - cos(theta1) * sin(theta2) * sin(theta3)) * ...
%     cos(theta4) + (-cos(theta1) * cos(theta2) * sin(theta3) - cos(theta1) * ...
%     sin(theta2) * cos(theta3)) * sin(theta4)) * sin(theta5) + 0.082 * ...
%     sin(theta1) * cos(theta5) + 0.093 * (cos(theta1) * cos(theta2) * ...
%     cos(theta3) - cos(theta1) * sin(theta2) * sin(theta3)) * sin(theta4) - ...
%     0.093 * (-cos(theta1) * cos(theta2) * sin(theta3) - cos(theta1) * ...
%     sin(theta2) * cos(theta3)) * cos(theta4) + 0.109 * sin(theta1) - ...
%     0.39243 * cos(theta1) * cos(theta2) * cos(theta3) + 0.39243 * ...
%     cos(theta1) * sin(theta2) * sin(theta3) - 0.425 * cos(theta1) * cos(theta2); ...
%     (((sin(theta1) * cos(theta2) * cos(theta3) - sin(theta1) * sin(theta2) * ...
%     sin(theta3)) * cos(theta4) + (-sin(theta1) * cos(theta2) * sin(theta3) - ...
%     sin(theta1) * sin(theta2) * cos(theta3)) * sin(theta4)) * cos(theta5) - ...
%     cos(theta1) * sin(theta5)) * cos(theta6) + (-(sin(theta1) * cos(theta2) * ...
%     cos(theta3) - sin(theta1) * sin(theta2) * sin(theta3)) * sin(theta4) + ...
%     (-sin(theta1) * cos(theta2) * sin(theta3) - sin(theta1) * sin(theta2) * ...
%     cos(theta3)) * cos(theta4)) * sin(theta6) -(((sin(theta1) * cos(theta2) *...
%     cos(theta3) - sin(theta1) * sin(theta2) * sin(theta3)) * cos(theta4) + ...
%     (-sin(theta1) * cos(theta2) * sin(theta3) - sin(theta1) * sin(theta2) * ...
%     cos(theta3)) * sin(theta4)) * cos(theta5) - cos(theta1) * sin(theta5)) * ...
%     sin(theta6) + (-(sin(theta1) * cos(theta2) * cos(theta3) - sin(theta1) * ...
%     sin(theta2) * sin(theta3)) * sin(theta4) + (-sin(theta1) * cos(theta2) * ...
%     sin(theta3) - sin(theta1) * sin(theta2) * cos(theta3)) * cos(theta4)) * ...
%     cos(theta6) -((sin(theta1) * cos(theta2) * cos(theta3) - sin(theta1) * ...
%     sin(theta2) * sin(theta3)) * cos(theta4) + (-sin(theta1) * cos(theta2) * ...
%     sin(theta3) - sin(theta1) * sin(theta2) * cos(theta3)) * sin(theta4)) *...
%      sin(theta5) - cos(theta1) * cos(theta5) -0.082 * ((sin(theta1) * ...
%     cos(theta2) * cos(theta3) - sin(theta1) * sin(theta2) * sin(theta3)) * ...
%     cos(theta4) + (-sin(theta1) * cos(theta2) * sin(theta3) - sin(theta1) * ...
%     sin(theta2) * cos(theta3)) * sin(theta4)) * sin(theta5) - 0.082 * ...
%     cos(theta1) * cos(theta5) + 0.093 * (sin(theta1) * cos(theta2) * ...
%     cos(theta3) - sin(theta1) * sin(theta2) * sin(theta3)) * sin(theta4) - ...
%     0.093 * (-sin(theta1) * cos(theta2) * sin(theta3) - sin(theta1) * ...
%     sin(theta2) * cos(theta3)) * cos(theta4) - 0.109 * cos(theta1) - ...
%     0.39243 * sin(theta1) * cos(theta2) * cos(theta3) + 0.39243 * ...
%     sin(theta1) * sin(theta2) * sin(theta3) - 0.425 * sin(theta1) * ...
%     cos(theta2); ((sin(theta2) * cos(theta3) + cos(theta2) * sin(theta3)) ...
%     * cos(theta4) + (-sin(theta2) * sin(theta3) + cos(theta2) * cos(theta3)) ...
%     * sin(theta4)) * cos(theta5) * cos(theta6) + (-(sin(theta2) * cos(theta3) ...
%     + cos(theta2) * sin(theta3)) * sin(theta4) + (-sin(theta2) * sin(theta3) ...
%     + cos(theta2) * cos(theta3)) * cos(theta4)) * sin(theta6) -((sin(theta2) ...
%     * cos(theta3) + cos(theta2) * sin(theta3)) * cos(theta4) + (-sin(theta2) ...
%     * sin(theta3) + cos(theta2) * cos(theta3)) * sin(theta4)) * cos(theta5) ...
%     * sin(theta6) + (-(sin(theta2) * cos(theta3) + cos(theta2) * sin(theta3)) ...
%     * sin(theta4) + (-sin(theta2) * sin(theta3) + cos(theta2) * cos(theta3)) ...
%     * cos(theta4)) * cos(theta6) -((sin(theta2) * cos(theta3) + cos(theta2) ...
%     * sin(theta3)) * cos(theta4) + (-sin(theta2) * sin(theta3) + cos(theta2) ...
%     * cos(theta3)) * sin(theta4)) * sin(theta5) 0.0892 - 0.082 * ...
%     ((sin(theta2) * cos(theta3) + cos(theta2) * sin(theta3)) * cos(theta4) ...
%     + (-sin(theta2) * sin(theta3) + cos(theta2) * cos(theta3)) * sin(theta4)) ...
%     * sin(theta5) + 0.093 * (sin(theta2) * cos(theta3) + cos(theta2) * ...
%     sin(theta3)) * sin(theta4) - 0.093 * (-sin(theta2) * sin(theta3) + ...
%     cos(theta2) * cos(theta3)) * cos(theta4) - 0.39243 * sin(theta2) * ...
%     cos(theta3) - 0.39243 * cos(theta2) * sin(theta3) - 0.425 * sin(theta2); ...
%     0 0 0 1;];

R = T(1:3,1:3);
d = T(1:3,4);

end

== matlab function JointSpaceControl_BestInertia/Forward & Velocity Kinematics Joint -> Tool Geometric Jacobian/base_tool_transformation_matrix ==
  data: d output; q input; R output
function [d, R]   = base_tool_transformation(q)
% BASE_TOOL_TRANSFORMATION - Transformationmatrix from Base to Tool.
%  Calculates the Base-Tool Transformation matrix based on the current
%  joint positions and returns the rotation matrix and the displacement
%  vector.

theta1 = q(1);
theta2 = q(2);
theta3 = q(3);
theta4 = q(4);
theta5 = q(5);
theta6 = q(6);

T = [(((cos(theta1) * cos(theta2) * cos(theta3) - cos(theta1) * sin(theta2) ...
    * sin(theta3)) * cos(theta4) + (-cos(theta1) * cos(theta2) * sin(theta3) ...
    - cos(theta1) * sin(theta2) * cos(theta3)) * sin(theta4)) * cos(theta5) ...
    + sin(theta1) * sin(theta5)) * cos(theta6) + (-(cos(theta1) * cos(theta2) ...
    * cos(theta3) - cos(theta1) * sin(theta2) * sin(theta3)) * sin(theta4) + ...
    (-cos(theta1) * cos(theta2) * sin(theta3) - cos(theta1) * sin(theta2) * ...
    cos(theta3)) * cos(theta4)) * sin(theta6) -(((cos(theta1) * cos(theta2) * ...
    cos(theta3) - cos(theta1) * sin(theta2) * sin(theta3)) * cos(theta4) + ...
    (-cos(theta1) * cos(theta2) * sin(theta3) - cos(theta1) * sin(theta2) * ...
    cos(theta3)) * sin(theta4)) * cos(theta5) + sin(theta1) * sin(theta5)) * ...
    sin(theta6) + (-(cos(theta1) * cos(theta2) * cos(theta3) - cos(theta1) * ...
    sin(theta2) * sin(theta3)) * sin(theta4) + (-cos(theta1) * cos(theta2) * ...
    sin(theta3) - cos(theta1) * sin(theta2) * cos(theta3)) * cos(theta4)) * ...
    cos(theta6) -((cos(theta1) * cos(theta2) * cos(theta3) - cos(theta1) * ...
    sin(theta2) * sin(theta3)) * cos(theta4) + (-cos(theta1) * cos(theta2) * ...
    sin(theta3) - cos(theta1) * sin(theta2) * cos(theta3)) * sin(theta4)) * ...
    sin(theta5) + sin(theta1) * cos(theta5) -0.082 * ((cos(theta1) * ...
    cos(theta2) * cos(theta3) - cos(theta1) * sin(theta2) * sin(theta3)) * ...
    cos(theta4) + (-cos(theta1) * cos(theta2) * sin(theta3) - cos(theta1) * ...
    sin(theta2) * cos(theta3)) * sin(theta4)) * sin(theta5) + 0.082 * ...
    sin(theta1) * cos(theta5) + 0.093 * (cos(theta1) * cos(theta2) * ...
    cos(theta3) - cos(theta1) * sin(theta2) * sin(theta3)) * sin(theta4) - ...
    0.093 * (-cos(theta1) * cos(theta2) * sin(theta3) - cos(theta1) * ...
    sin(theta2) * cos(theta3)) * cos(theta4) + 0.109 * sin(theta1) - ...
    0.39243 * cos(theta1) * cos(theta2) * cos(theta3) + 0.39243 * ...
    cos(theta1) * sin(theta2) * sin(theta3) - 0.425 * cos(theta1) * cos(theta2); ...
    (((sin(theta1) * cos(theta2) * cos(theta3) - sin(theta1) * sin(theta2) * ...
    sin(theta3)) * cos(theta4) + (-sin(theta1) * cos(theta2) * sin(theta3) - ...
    sin(theta1) * sin(theta2) * cos(theta3)) * sin(theta4)) * cos(theta5) - ...
    cos(theta1) * sin(theta5)) * cos(theta6) + (-(sin(theta1) * cos(theta2) * ...
    cos(theta3) - sin(theta1) * sin(theta2) * sin(theta3)) * sin(theta4) + ...
    (-sin(theta1) * cos(theta2) * sin(theta3) - sin(theta1) * sin(theta2) * ...
    cos(theta3)) * cos(theta4)) * sin(theta6) -(((sin(theta1) * cos(theta2) *...
    cos(theta3) - sin(theta1) * sin(theta2) * sin(theta3)) * cos(theta4) + ...
    (-sin(theta1) * cos(theta2) * sin(theta3) - sin(theta1) * sin(theta2) * ...
    cos(theta3)) * sin(theta4)) * cos(theta5) - cos(theta1) * sin(theta5)) * ...
    sin(theta6) + (-(sin(theta1) * cos(theta2) * cos(theta3) - sin(theta1) * ...
    sin(theta2) * sin(theta3)) * sin(theta4) + (-sin(theta1) * cos(theta2) * ...
    sin(theta3) - sin(theta1) * sin(theta2) * cos(theta3)) * cos(theta4)) * ...
    cos(theta6) -((sin(theta1) * cos(theta2) * cos(theta3) - sin(theta1) * ...
    sin(theta2) * sin(theta3)) * cos(theta4) + (-sin(theta1) * cos(theta2) * ...
    sin(theta3) - sin(theta1) * sin(theta2) * cos(theta3)) * sin(theta4)) *...
     sin(theta5) - cos(theta1) * cos(theta5) -0.082 * ((sin(theta1) * ...
    cos(theta2) * cos(theta3) - sin(theta1) * sin(theta2) * sin(theta3)) * ...
    cos(theta4) + (-sin(theta1) * cos(theta2) * sin(theta3) - sin(theta1) * ...
    sin(theta2) * cos(theta3)) * sin(theta4)) * sin(theta5) - 0.082 * ...
    cos(theta1) * cos(theta5) + 0.093 * (sin(theta1) * cos(theta2) * ...
    cos(theta3) - sin(theta1) * sin(theta2) * sin(theta3)) * sin(theta4) - ...
    0.093 * (-sin(theta1) * cos(theta2) * sin(theta3) - sin(theta1) * ...
    sin(theta2) * cos(theta3)) * cos(theta4) - 0.109 * cos(theta1) - ...
    0.39243 * sin(theta1) * cos(theta2) * cos(theta3) + 0.39243 * ...
    sin(theta1) * sin(theta2) * sin(theta3) - 0.425 * sin(theta1) * ...
    cos(theta2); ((sin(theta2) * cos(theta3) + cos(theta2) * sin(theta3)) ...
    * cos(theta4) + (-sin(theta2) * sin(theta3) + cos(theta2) * cos(theta3)) ...
    * sin(theta4)) * cos(theta5) * cos(theta6) + (-(sin(theta2) * cos(theta3) ...
    + cos(theta2) * sin(theta3)) * sin(theta4) + (-sin(theta2) * sin(theta3) ...
    + cos(theta2) * cos(theta3)) * cos(theta4)) * sin(theta6) -((sin(theta2) ...
    * cos(theta3) + cos(theta2) * sin(theta3)) * cos(theta4) + (-sin(theta2) ...
    * sin(theta3) + cos(theta2) * cos(theta3)) * sin(theta4)) * cos(theta5) ...
    * sin(theta6) + (-(sin(theta2) * cos(theta3) + cos(theta2) * sin(theta3)) ...
    * sin(theta4) + (-sin(theta2) * sin(theta3) + cos(theta2) * cos(theta3)) ...
    * cos(theta4)) * cos(theta6) -((sin(theta2) * cos(theta3) + cos(theta2) ...
    * sin(theta3)) * cos(theta4) + (-sin(theta2) * sin(theta3) + cos(theta2) ...
    * cos(theta3)) * sin(theta4)) * sin(theta5) 0.0892 - 0.082 * ...
    ((sin(theta2) * cos(theta3) + cos(theta2) * sin(theta3)) * cos(theta4) ...
    + (-sin(theta2) * sin(theta3) + cos(theta2) * cos(theta3)) * sin(theta4)) ...
    * sin(theta5) + 0.093 * (sin(theta2) * cos(theta3) + cos(theta2) * ...
    sin(theta3)) * sin(theta4) - 0.093 * (-sin(theta2) * sin(theta3) + ...
    cos(theta2) * cos(theta3)) * cos(theta4) - 0.39243 * sin(theta2) * ...
    cos(theta3) - 0.39243 * cos(theta2) * sin(theta3) - 0.425 * sin(theta2); ...
    0 0 0 1;];

R = T(1:3,1:3);
d = T(1:3,4);

end

== matlab function JointSpaceControl_BestInertia/Forward & Velocity Kinematics Joint -> Tool Geometric Jacobian/Euler -> R ==
  data: theta input; phi input; R output; psi input
function R   = Euler_angle_to_R(theta, phi, psi)
%R_TO_EULER_ANGLE Transform rotation matrix to euler-angle format, where
%the rotation happens around ZYZ, with R_ZYZ = R_Z,phi*R_Y,theta*R_Z,psi

r_11 = cos(phi)*cos(theta)*cos(psi)-sin(phi)*sin(psi);
r_12 = -cos(phi)*cos(theta)*sin(psi)-sin(phi)*cos(psi);
r_13 = cos(phi)*sin(theta);

r_21 = sin(phi)*cos(theta)*cos(psi) + cos(phi)*sin(psi);
r_22 = -sin(phi)*cos(theta)*sin(psi)+cos(phi)*cos(psi);
r_23 = sin(phi)*sin(theta);

r_31 = -sin(theta)*cos(psi);
r_32 = sin(theta)*sin(psi);
r_33 = cos(theta);

R = [r_11, r_12, r_13; ...
     r_21, r_22, r_23; ...
     r_31, r_32, r_33];
end

== matlab function JointSpaceControl_BestInertia/Forward & Velocity Kinematics Joint -> Tool Geometric Jacobian/Joints -> End-Effector/from_me2 ==
  data: J_a input; dJ_a input; dq input; ddq input; ddX output
function ddX     = ddX(J_a, dJ_a, dq, ddq)
% ANALYTICAL JACOBIAN - Jacobian from Base to Tool.
%  Calculates the analytical Jacobian, based on the Euler angle transform
%  representation.

ddX = J_a*ddq + dJ_a*dq;

end

== matlab function JointSpaceControl_BestInertia/Forward & Velocity Kinematics Joint -> Tool Geometric Jacobian/Joints -> End-Effector/from_me4 ==
  data: J_a input; dq input; dX output
function dX     = dX(J_a, dq)
% ANALYTICAL JACOBIAN - Jacobian from Base to Tool.
%  Calculates the analytical Jacobian, based on the Euler angle transform
%  representation.

dX = J_a*dq;

end

== matlab function JointSpaceControl_BestInertia/Forward & Velocity Kinematics Joint -> Tool Geometric Jacobian/End-Effector -> Joints/from_me5 ==
  data: J_a input; dq output; dX input
function dq     = dq(J_a, dX)
% ANALYTICAL JACOBIAN - Jacobian from Base to Tool.
%  Calculates the analytical Jacobian, based on the Euler angle transform
%  representation.

dq = J_a\dX;

end

== matlab function JointSpaceControl_BestInertia/Forward & Velocity Kinematics Joint -> Tool Geometric Jacobian/End-Effector -> Joints/from_me6 ==
  data: J_a input; dJ_a input; ddX input; dq input; ddq output
function ddq     = ddq(J_a, dJ_a, ddX, dq)
% ANALYTICAL JACOBIAN - Jacobian from Base to Tool.
%  Calculates the analytical Jacobian, based on the Euler angle transform
%  representation.

% ddq = inv(J_a)*(ddX - dJ_a*dq);


    ddq = J_a\(ddX - dJ_a*dq);


end

== matlab function JointSpaceControl_BestInertia/Forward & Velocity Kinematics Joint -> Tool Geometric Jacobian/rank(J) ==
  data: J input; rank_J output
function rank_J   = rank_J(J)
%Calculate the rank of a matrix J.

rank_J = svd(J);
end

== matlab function JointSpaceControl_BestInertia/Inverse Dynamics M, C, g1/ur5_invDynamics ==
  data: a_q input; M input; G input; CDq input; tau output
function tau = ur5_invDynamics(a_q, M, G, CDq)
%#codegen
%Returns the torque that must be applied to the robot given the desired
%position, velocity and acceleration
tau = M*a_q + CDq + G;

== matlab function JointSpaceControl_BestInertia/Robot UR5 M, C, g/ur5_dynamics ==
  data: q input; dq input; tau input; ddq output
function ddq = ur5_dynamics( q, dq, tau )
%#codegen
%Returns the acceleration of the manipulator based on its dynamics
[ M, G, CDq ] = ur5_matrices( q, dq );

ddq = M \ (tau - CDq - G);

== matlab function JointSpaceControl_BestInertia/Inverse Dynamics M, C, g/MATLAB Function6 ==
  data: a_q input; M input; G input; CDq input; tau output; tau_M output; tau_CDq output; tau_G output
function [tau, tau_M, tau_CDq, tau_G] = ur5_invDynamics(a_q, M, G, CDq)
%#codegen
%Returns the torque that must be applied to the robot given the desired
%position, velocity and acceleration
tau = M*a_q + CDq + G;
tau_M = M*a_q;
tau_CDq = CDq;
tau_G = G;
